simulink model "mass"  (R2022a)
settings: Solver=VariableStepAuto  StartTime=0.0  StopTime=5  MaxStep=0.025  RelTol=1e-3  AbsTol=1e-3
PostLoadFcn:
  | m = 3.600 %Kg
  | k = 400 %N/m
  | b = 10 %N/(m/s)
  | x0 = 1 %m
settings Model: Creator=mluser  LastModifiedBy=mluser

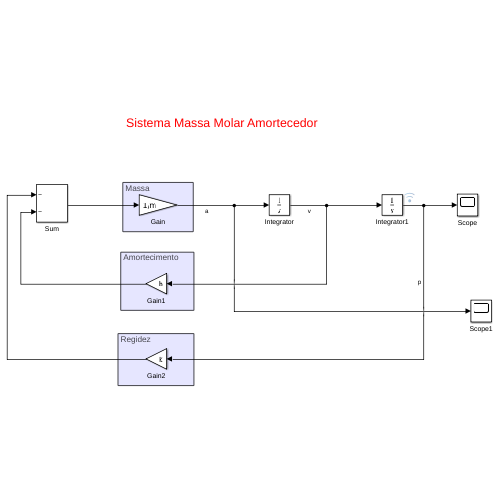
[thumbnail: Simulink's stored preview of the top-level diagram]
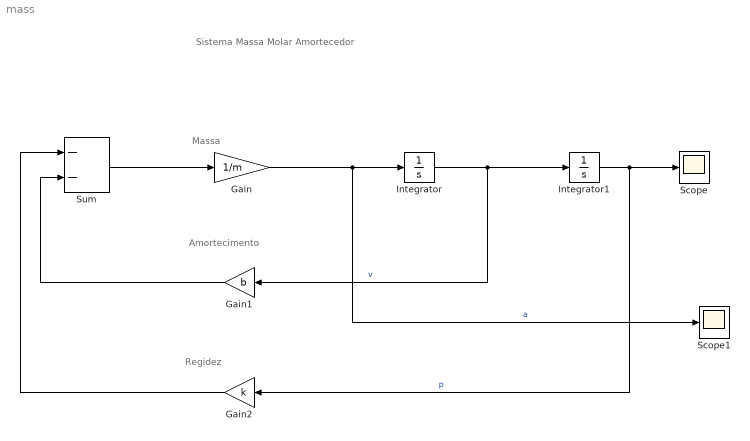
== system mass ==
  note: Regidez
  note: Amortecimento
  note: Massa
  note: Sistema Massa Molar Amortecedor
  Gain : Gain  Gain=1/m  ParamDataTypeStr=Inherit: Same as input
  Gain1 : Gain  Gain=b  ParamDataTypeStr=Inherit: Same as input
  Gain2 : Gain  Gain=k  ParamDataTypeStr=Inherit: Same as input
  Integrator : Integrator
  Integrator1 : Integrator  InitialCondition=1
  Scope : Scope
  Scope1 : Scope
  Sum : Sum  Inputs=--
  wires:
  Sum/1 -> Gain/1
  Gain/1 -> Scope1/1, Integrator/1  "a"
  Integrator/1 -> Gain1/1, Integrator1/1  "v"
  Integrator1/1 -> Gain2/1, Scope/1  "p"
  Gain2/1 -> Sum/1
  Gain1/1 -> Sum/2
